simulink library "xrbsDSP_r3"  (Simulink 5.0)
undefined symbols (not defined in the file or in its folder): FIR1, Ft, mem
libraries: xbsIndex_r3 x329
(part 3 of 4)

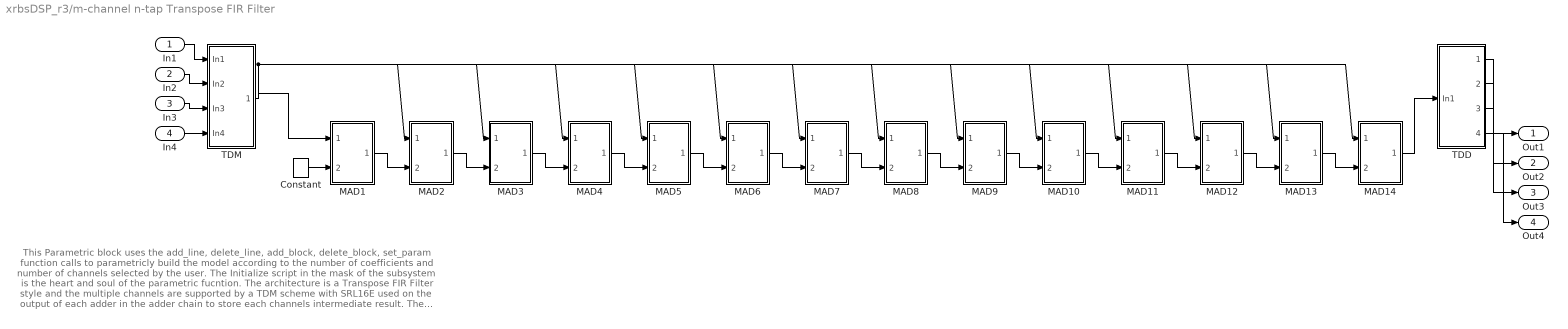
== system xrbsDSP_r3/m-channel n-tap Transpose FIR Filter ==
  note: This Parametric block uses the add_line, delete_line, add_block, delete_block, set_param function calls to parametricly
      | build the model according to the number of coefficients and number of channels selected by the user. The Initialize script in
      | the mask of the subsystem is the heart and soul of the parametric fucntion.
      |
      | The architecture is a Transpose FIR Filter style and the multiple channels are supported by a TDM scheme with SRL16E used
      | on the output of each adder in the adder chain to store each channels intermediate result. The clock will always be N channels
      | times faster that the input sample rate.
  In1 : Inport
  In2 : Inport  Port=2
  In3 : Inport  Port=3
  In4 : Inport  Port=4
  Constant : xbsIndex_r3/Constant  const=0  arith_type=Unsigned  n_bits=1  bin_pt=0  explicit_period=off  period=1  dbl_ovrd=off
  MAD1 : Subsystem  mask(MAD Block){coef=coef_array(1), coef_bitwidth=coef_bitwidth, coef_binpt=coef_binpt, channels=channels}
      mask prompts: coef "Coefficient Value"; coef_bitwidth "Coefficient Bit Width"; coef_binpt "Coefficient Binary Point"; channels "Number of Channels"
  MAD10 : Subsystem  mask(MAD Block){coef=coef_array(10), coef_bitwidth=coef_bitwidth, coef_binpt=coef_binpt, channels=channels}
      mask prompts: coef "Coefficient Value"; coef_bitwidth "Coefficient Bit Width"; coef_binpt "Coefficient Binary Point"; channels "Number of Channels"
  MAD11 : Subsystem  mask(MAD Block){coef=coef_array(11), coef_bitwidth=coef_bitwidth, coef_binpt=coef_binpt, channels=channels}
      mask prompts: coef "Coefficient Value"; coef_bitwidth "Coefficient Bit Width"; coef_binpt "Coefficient Binary Point"; channels "Number of Channels"
  MAD12 : Subsystem  mask(MAD Block){coef=coef_array(12), coef_bitwidth=coef_bitwidth, coef_binpt=coef_binpt, channels=channels}
      mask prompts: coef "Coefficient Value"; coef_bitwidth "Coefficient Bit Width"; coef_binpt "Coefficient Binary Point"; channels "Number of Channels"
  MAD13 : Subsystem  mask(MAD Block){coef=coef_array(13), coef_bitwidth=coef_bitwidth, coef_binpt=coef_binpt, channels=channels}
      mask prompts: coef "Coefficient Value"; coef_bitwidth "Coefficient Bit Width"; coef_binpt "Coefficient Binary Point"; channels "Number of Channels"
  MAD14 : Subsystem  mask(MAD Block){coef=coef_array(14), coef_bitwidth=coef_bitwidth, coef_binpt=coef_binpt, channels=channels}
      mask prompts: coef "Coefficient Value"; coef_bitwidth "Coefficient Bit Width"; coef_binpt "Coefficient Binary Point"; channels "Number of Channels"
  MAD2 : Subsystem  mask(MAD Block){coef=coef_array(2), coef_bitwidth=coef_bitwidth, coef_binpt=coef_binpt, channels=channels}
      mask prompts: coef "Coefficient Value"; coef_bitwidth "Coefficient Bit Width"; coef_binpt "Coefficient Binary Point"; channels "Number of Channels"
  MAD3 : Subsystem  mask(MAD Block){coef=coef_array(3), coef_bitwidth=coef_bitwidth, coef_binpt=coef_binpt, channels=channels}
      mask prompts: coef "Coefficient Value"; coef_bitwidth "Coefficient Bit Width"; coef_binpt "Coefficient Binary Point"; channels "Number of Channels"
  MAD4 : Subsystem  mask(MAD Block){coef=coef_array(4), coef_bitwidth=coef_bitwidth, coef_binpt=coef_binpt, channels=channels}
      mask prompts: coef "Coefficient Value"; coef_bitwidth "Coefficient Bit Width"; coef_binpt "Coefficient Binary Point"; channels "Number of Channels"
  MAD5 : Subsystem  mask(MAD Block){coef=coef_array(5), coef_bitwidth=coef_bitwidth, coef_binpt=coef_binpt, channels=channels}
      mask prompts: coef "Coefficient Value"; coef_bitwidth "Coefficient Bit Width"; coef_binpt "Coefficient Binary Point"; channels "Number of Channels"
  MAD6 : Subsystem  mask(MAD Block){coef=coef_array(6), coef_bitwidth=coef_bitwidth, coef_binpt=coef_binpt, channels=channels}
      mask prompts: coef "Coefficient Value"; coef_bitwidth "Coefficient Bit Width"; coef_binpt "Coefficient Binary Point"; channels "Number of Channels"
  MAD7 : Subsystem  mask(MAD Block){coef=coef_array(7), coef_bitwidth=coef_bitwidth, coef_binpt=coef_binpt, channels=channels}
      mask prompts: coef "Coefficient Value"; coef_bitwidth "Coefficient Bit Width"; coef_binpt "Coefficient Binary Point"; channels "Number of Channels"
  MAD8 : Subsystem  mask(MAD Block){coef=coef_array(8), coef_bitwidth=coef_bitwidth, coef_binpt=coef_binpt, channels=channels}
      mask prompts: coef "Coefficient Value"; coef_bitwidth "Coefficient Bit Width"; coef_binpt "Coefficient Binary Point"; channels "Number of Channels"
  MAD9 : Subsystem  mask(MAD Block){coef=coef_array(9), coef_bitwidth=coef_bitwidth, coef_binpt=coef_binpt, channels=channels}
      mask prompts: coef "Coefficient Value"; coef_bitwidth "Coefficient Bit Width"; coef_binpt "Coefficient Binary Point"; channels "Number of Channels"
  TDD : Subsystem
      mask Type: TDD
      mask Description: Multi-Channel Time Division DeMultiplexer
  TDM : Subsystem
  Out1 : Outport
  Out2 : Outport  Port=2
  Out3 : Outport  Port=3
  Out4 : Outport  Port=4
  wires:
  Constant/1 -> MAD1/2(In2)
  TDM/1(Out1) -> MAD1/1(In1), MAD2/1(In1), MAD3/1(In1), MAD4/1(In1), MAD5/1(In1), MAD6/1(In1), MAD7/1(In1), MAD8/1(In1), MAD9/1(In1), MAD10/1(In1), MAD11/1(In1), MAD12/1(In1), MAD13/1(In1), MAD14/1(In1)
  In1/1 -> TDM/1(In1)
  MAD1/1(Out1) -> MAD2/2(In2)
  MAD2/1(Out1) -> MAD3/2(In2)
  MAD3/1(Out1) -> MAD4/2(In2)
  MAD4/1(Out1) -> MAD5/2(In2)
  MAD5/1(Out1) -> MAD6/2(In2)
  MAD6/1(Out1) -> MAD7/2(In2)
  MAD7/1(Out1) -> MAD8/2(In2)
  MAD8/1(Out1) -> MAD9/2(In2)
  MAD9/1(Out1) -> MAD10/2(In2)
  MAD10/1(Out1) -> MAD11/2(In2)
  MAD11/1(Out1) -> MAD12/2(In2)
  MAD12/1(Out1) -> MAD13/2(In2)
  MAD13/1(Out1) -> MAD14/2(In2)
  MAD14/1(Out1) -> TDD/1(In1)
  TDD/1(Out1) -> Out1/1
  TDD/2(Out2) -> Out2/1
  TDD/3(Out3) -> Out3/1
  TDD/4(Out4) -> Out4/1
  In2/1 -> TDM/2(In2)
  In3/1 -> TDM/3(In3)
  In4/1 -> TDM/4(In4)

== system xrbsDSP_r3/n-tap Dual Port Memory MAC FIR Filter ==
  note: The 'Address Control' subsystem
      | provides the necessary address
      | logic for the Dual Port RAM.
      | The control logic creates a cyclic
      | RAM buffer for port A (data buffer)
      | to create the required shifting
      | effect.
  note: A Dual Port Block RAM implements the input data buffer.
      | The address port runs n times faster than the data port,
      | where n is the number of filter taps.
      |
      | The filter coefficients are also stored in the same Dual Port
      | Block RAM and are output from port B.
  note: A down sampler reduces the capture register
      | sample period to the output sample period.
      | The block is configured with latency to obtain  the
      | most efficient hardware implementation.  The down
      | sampling rate is equal to the coefficient array length.
  note: A capture register is required for streaming
      | operation, since the MAC engine reloads its
      | accumulator with an incoming sample after
      | computing the last partial product for an output
      | sample.
  note: As configured, the filter occupies 84 slices, 1 dedicated multiplier,
      | and 1 block memory.  The maximum clock frequency is approximately
      | 180 MHz in a Xilinx xc2vp2-7 part (advanced speeds files 1.69, ISE
      | 5.1.03i software).
  din : Inport
  Accumulator : xbsIndex_r3/Accumulator  n_bits=accum_bit_width  overflow=Wrap  operation=Add  scale=1  explicit_period=off  period=1  rst=on  hasbypass=on  en=off  dbl_ovrd=off  show_param=off  gen_core=on  use_rpm=off
      settings: xl_area=[0, 0, 0, 0, 0, 0, 0]
  Address Control : Subsystem
  Capture Register : xbsIndex_r3/Register  init=0  reg_only_valid=on  explicit_period=off  period=1  rst=off  en=on  out_en=off  dbl_ovrd=off  show_param=off
      settings: xl_area=[0, 0, 0, 0, 0, 0, 0]
  Delay : xbsIndex_r3/Delay  latency=3  reg_retiming=off  explicit_period=off  period=1  en=off  accept_only_valid=off  init_zero=on  dbl_ovrd=off  show_param=off
      settings: xl_area=[0, 0, 0, 0, 0, 0, 0]
  Down Sample : xbsIndex_r3/Down Sample  sample_ratio=length(coef)  sample_phase="Last Value of Frame  (most efficient)"  latency=1  en=off  dbl_ovrd=off  show_param=off
      settings: xl_area=[0, 0, 0, 0, 0, 0, 0]
  Dual Port RAM : Subsystem
  Mult : xbsIndex_r3/Mult  precision=Full  arith_type="Signed  (2's comp)"  n_bits=8  bin_pt=2  quantization=Truncate  overflow=Wrap  latency=2  explicit_period=off  period=1/(22050*length(coef))  en=off  dbl_ovrd=off  show_param=off  mult_type=Parallel  oversample=2  use_embedded=on  pipeline=on  use_rpm=off  placement_style=Rectangular Shape  gen_core=on
      settings: xl_area=[0, 0, 0, 0, 0, 0, 0]
  dout : Outport
  wires:
  Delay/1 -> Accumulator/2, Capture Register/2
  Address Control/4(rst) -> Delay/1
  Dual Port RAM/2(dout_b) -> Mult/2
  Dual Port RAM/1(dout_a) -> Mult/1
  din/1 -> Dual Port RAM/1(din)
  Address Control/3(coef_addr) -> Dual Port RAM/4(coef_addr)
  Address Control/2(we) -> Dual Port RAM/3(we)
  Address Control/1(data_addr) -> Dual Port RAM/2(data_addr)
  Capture Register/1 -> Down Sample/1
  Accumulator/1 -> Capture Register/1
  Down Sample/1 -> dout/1
  Mult/1 -> Accumulator/1

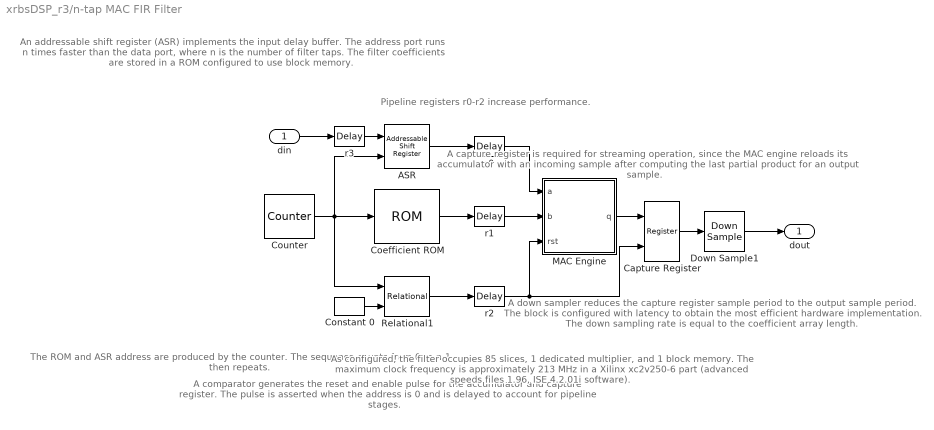
== system xrbsDSP_r3/n-tap MAC FIR Filter ==
  note: A capture register is required for streaming
      | operation, since the MAC engine reloads its
      | accumulator with an incoming sample after
      | computing the last partial product for an output
      | sample.
  note: Pipeline registers r0-r2
      | increase performance.
  note: An addressable shift register (ASR)
      | implements the input delay buffer.
      | The address port runs n times faster
      | than the data port, where n is the number
      | of filter taps.
      |
      | The filter coefficients are stored in a ROM
      | configured to use block memory.
  note: The ROM and ASR
      | address are produced
      | by the counter.  The
      | sequence counts from
      | 0 to n-1, then repeats.
  note: A comparator generates
      | the reset and enable
      | pulse for the accumulator
      | and capture register.  The
      | pulse is asserted when
      | the address is 0 and is
      | delayed to account for
      | pipeline stages.
  note: As configured, the  filter occupies 85 slices, 1 dedicated multiplier, and
      | 1 block memory.  The maximum clock frequency is approximately
      | 213 MHz in a Xilinx xc2v250-6 part (advanced speeds files 1.96, ISE
      | 4.2.01i software).
  note: A down sampler reduces the capture register
      | sample period to the output sample period.
      | The block is configured with latency to obtain  the
      | most efficient hardware implementation.  The down
      | sampling rate is equal to the coefficient array length.
  din : Inport
  ASR : xbsIndex_r3/Addressable Shift Register  infer_latency=on  depth=2  initVector=0  explicit_period=off  period=1  accept_only_valid=off  en=off  dbl_ovrd=off  show_param=off  use_rpm=off  gen_core=off
      settings: xl_area=[0, 0, 0, 0, 0, 0, 0]
  Capture Register : xbsIndex_r3/Register  init=0  reg_only_valid=on  explicit_period=off  period=1  rst=off  en=on  out_en=off  dbl_ovrd=off  show_param=off
      settings: xl_area=[0, 0, 0, 0, 0, 0, 0]
  Coefficient ROM : xbsIndex_r3/ROM  depth=length(coef)  initVector=coef  arith_type="Signed  (2's comp)"  n_bits=coef_n_bits  bin_pt=coef_bin_pt  latency=1  init_zero=on  explicit_period=off  period=1  rst=off  init_reg=0  en=off  dbl_ovrd=off  show_param=off  distributed_mem=off  use_rpm=off  gen_core=on
      settings: xl_area=[0, 0, 0, 0, 0, 0, 0]
  Constant 0 : xbsIndex_r3/Constant  const=0  arith_type=Unsigned  n_bits=1  bin_pt=0  explicit_period=off  period=1  dbl_ovrd=off
  Counter : xbsIndex_r3/Counter  cnt_type=Count Limited  n_bits=ceil(log2(length(coef)))  bin_pt=0  arith_type=Unsigned  start_count=0  cnt_to=length(coef)-1  cnt_by_val=1  operation=Up  explicit_period=on  period=smpl_period/length(coef)  load_pin=off  rst=off  en=off  dbl_ovrd=off  show_param=off  use_rpm=on  gen_core=on
      settings: xl_area=[0, 0, 0, 0, 0, 0, 0]
  Down Sample1 : xbsIndex_r3/Down Sample  sample_ratio=length(coef)  sample_phase="Last Value of Frame  (most efficient)"  latency=1  en=off  dbl_ovrd=off  show_param=off
      settings: xl_area=[0, 0, 0, 0, 0, 0, 0]
  MAC Engine : Subsystem
  Relational1 : xbsIndex_r3/Relational  mode=a=b  latency=3  explicit_period=off  period=1  en=off  dbl_ovrd=off  show_param=off
      settings: xl_area=[0, 0, 0, 0, 0, 0, 0]
  r0 : xbsIndex_r3/Delay  latency=2  reg_retiming=off  explicit_period=off  period=1  en=off  accept_only_valid=off  init_zero=on  dbl_ovrd=off  show_param=off
      settings: xl_area=[0, 0, 0, 0, 0, 0, 0]
  r1 : xbsIndex_r3/Delay  latency=1  reg_retiming=off  explicit_period=off  period=1  en=off  accept_only_valid=off  init_zero=on  dbl_ovrd=off  show_param=off
      settings: xl_area=[0, 0, 0, 0, 0, 0, 0]
  r2 : xbsIndex_r3/Delay  latency=1  reg_retiming=off  explicit_period=off  period=1  en=off  accept_only_valid=off  init_zero=on  dbl_ovrd=off  show_param=off
      settings: xl_area=[0, 0, 0, 0, 0, 0, 0]
  r3 : xbsIndex_r3/Delay  latency=1  reg_retiming=off  explicit_period=off  period=1  en=off  accept_only_valid=off  init_zero=on  dbl_ovrd=off  show_param=off
      settings: xl_area=[0, 0, 0, 0, 0, 0, 0]
  dout : Outport
  wires:
  din/1 -> r3/1
  r1/1 -> MAC Engine/2(b)
  r0/1 -> MAC Engine/1(a)
  ASR/1 -> r0/1
  Counter/1 -> Coefficient ROM/1, ASR/2, Relational1/1
  r3/1 -> ASR/1
  Constant 0/1 -> Relational1/2
  Coefficient ROM/1 -> r1/1
  MAC Engine/1(q) -> Capture Register/1
  Down Sample1/1 -> dout/1
  Capture Register/1 -> Down Sample1/1
  Relational1/1 -> r2/1
  r2/1 -> Capture Register/2, MAC Engine/3(rst)

== system xrbsDSP_r3/2 Channel  Decimate by 2  MAC FIR Filter/2 Channel Accum ==
  d : Inport
  rst : Inport  Port=2
  AddSub : xbsIndex_r3/AddSub  mode=Addition  precision=User Defined  arith_type="Signed  (2's comp)"  n_bits=ceil(log2(coef_sum*(2^(bit_width-1))))+1  bin_pt=coef_bin_pt+bin_pt  quantization=Truncate  overflow=Wrap  latency=0  explicit_period=on  period=-1  use_carryin=off  use_carryout=off  en=off  dbl_ovrd=off  show_param=off  use_core=on  pipeline=off  use_rpm=off  gen_core=on
      settings: xl_area=[18 0 0 36 0 0 0]
  Delay : xbsIndex_r3/Delay  Orientation=left  latency=1  reg_retiming=off  explicit_period=off  period=1  en=off  accept_only_valid=off  init_zero=on  dbl_ovrd=off  show_param=off
      settings: xl_area=[18 36 0 0 0 0 0]
  Mux : xbsIndex_r3/Mux  inputs=2  precision=Full  arith_type="Signed  (2's comp)"  n_bits=8  bin_pt=2  quantization=Truncate  overflow=Wrap  latency=0  explicit_period=off  period=1  en=off  dbl_ovrd=off  show_param=off  mux_type=off  use_rpm=off  gen_core=on
      settings: xl_area=[36 0 0 36 0 0 0]
  Register : xbsIndex_r3/Register  init=0  reg_only_valid=off  explicit_period=off  period=1  rst=off  en=off  out_en=off  dbl_ovrd=off  show_param=off
      settings: xl_area=[18 36 0 0 0 0 0]
  q : Outport
  wires:
  Delay/1 -> AddSub/2
  Register/1 -> q/1, Delay/1
  Mux/1 -> Register/1
  AddSub/1 -> Mux/3
  rst/1 -> Mux/1
  d/1 -> Mux/2, AddSub/1

== system xrbsDSP_r3/2 Channel  Decimate by 2  MAC FIR Filter/2:1 Mux ==
  din1 : Inport
  din2 : Inport  Port=2
  Counter : xbsIndex_r3/Counter  cnt_type=Free Running  n_bits=1  bin_pt=0  arith_type=Unsigned  start_count=0  cnt_to=Inf  cnt_by_val=1  operation=Up  explicit_period=off  period=Ts/2  load_pin=off  rst=off  en=off  dbl_ovrd=off  use_rpm=off  gen_core=on
      settings: xl_area=[2 1 0 1 0 0 0]
  Delay2 : xbsIndex_r3/Delay  latency=1  reg_retiming=off  explicit_period=off  period=1  en=off  accept_only_valid=off  init_zero=on  dbl_ovrd=off
      settings: xl_area=[0, 0, 0, 0, 0, 0, 0]
  Mux : xbsIndex_r3/Mux  inputs=2  precision=Full  arith_type="Signed  (2's comp)"  n_bits=8  bin_pt=2  quantization=Truncate  overflow=Wrap  latency=0  mux_type=off  explicit_period=off  period=1  en=off  dbl_ovrd=off  use_rpm=off  gen_core=on
      settings: xl_area=[0, 0, 0, 0, 0, 0, 0]
  Up Sample : xbsIndex_r3/Up Sample  sample_ratio=2  copy_samples=on  dbl_ovrd=off
      settings: xl_area=[0, 0, 0, 0, 0, 0, 0]
  Up Sample1 : xbsIndex_r3/Up Sample  sample_ratio=2  copy_samples=on  dbl_ovrd=off
      settings: xl_area=[0, 0, 0, 0, 0, 0, 0]
  Up Sample2 : xbsIndex_r3/Up Sample  sample_ratio=length(coef)/4  copy_samples=on  dbl_ovrd=off
      settings: xl_area=[0, 0, 0, 0, 0, 0, 0]
  dout : Outport
  wires:
  Up Sample2/1 -> dout/1
  din2/1 -> Up Sample1/1
  din1/1 -> Up Sample/1
  Delay2/1 -> Up Sample2/1
  Mux/1 -> Delay2/1
  Counter/1 -> Mux/1
  Up Sample1/1 -> Mux/3
  Up Sample/1 -> Mux/2

== system xrbsDSP_r3/2 Channel  Decimate by 2  MAC FIR Filter/Accum Control ==
  Constant1 : xbsIndex_r3/Constant  const=2  arith_type=Unsigned  n_bits=2  bin_pt=0  explicit_period=off  period=1  dbl_ovrd=off
  Constant4 : xbsIndex_r3/Constant  const=0  arith_type=Unsigned  n_bits=2  bin_pt=0  explicit_period=off  period=1  dbl_ovrd=off
  Constant5 : xbsIndex_r3/Constant  const=1  arith_type=Unsigned  n_bits=2  bin_pt=0  explicit_period=off  period=1  dbl_ovrd=off
  Counter : xbsIndex_r3/Counter  cnt_type=Free Running  n_bits=2  bin_pt=0  arith_type=Unsigned  start_count=0  cnt_to=Inf  cnt_by_val=1  operation=Up  explicit_period=off  period=Ts/2  load_pin=off  rst=off  en=off  dbl_ovrd=off  use_rpm=off  gen_core=on
      settings: xl_area=[1 2 0 2 0 0 0]
  Logical : xbsIndex_r3/Logical  logical_function=OR  inputs=2  precision=Full  arith_type=Unsigned  n_bits=8  bin_pt=2  align_bp=on  latency=0  explicit_period=off  period=1  en=off  dbl_ovrd=off
      settings: xl_area=[1 0 0 1 0 0 0]
  Relational1 : xbsIndex_r3/Relational  mode=a=b  latency=0  explicit_period=off  period=1  en=off  dbl_ovrd=off
      settings: xl_area=[2 0 0 1 0 0 0]
  Relational4 : xbsIndex_r3/Relational  mode=a=b  latency=0  explicit_period=off  period=1  en=off  dbl_ovrd=off
      settings: xl_area=[2 0 0 1 0 0 0]
  Relational5 : xbsIndex_r3/Relational  mode=a=b  latency=0  explicit_period=off  period=1  en=off  dbl_ovrd=off
      settings: xl_area=[2 0 0 1 0 0 0]
  rst : Outport
  en_a : Outport  Port=2
  en_b : Outport  Port=3
  wires:
  Relational1/1 -> en_b/1
  Constant1/1 -> Relational1/2
  Logical/1 -> rst/1
  Relational5/1 -> en_a/1, Logical/2
  Relational4/1 -> Logical/1
  Constant5/1 -> Relational5/2
  Constant4/1 -> Relational4/2
  Counter/1 -> Relational4/1, Relational1/1, Relational5/1

== system xrbsDSP_r3/2 Channel  Decimate by 2  MAC FIR Filter/Data Buffer ==
  din : Inport
  data_addr : Inport  Port=2
  en : Inport  Port=3
  coef_addr : Inport  Port=4
  ASR : xbsIndex_r3/Addressable Shift Register  infer_latency=on  depth=2  initVector=[0]  explicit_period=off  period=1  accept_only_valid=off  en=on  dbl_ovrd=off  use_rpm=off  gen_core=<empty>
      settings: xl_area=[0, 0, 0, 0, 0, 0, 0]
  Delay1 : xbsIndex_r3/Delay  latency=1  reg_retiming=off  explicit_period=off  period=1  en=off  accept_only_valid=off  init_zero=on  dbl_ovrd=off
      settings: xl_area=[0, 0, 0, 0, 0, 0, 0]
  ROM : xbsIndex_r3/ROM  depth=length(coef)  initVector=coef  arith_type="Signed  (2's comp)"  n_bits=coef_bit_width  bin_pt=coef_bin_pt  latency=1  distributed_mem=off  init_zero=on  explicit_period=off  period=1  rst=off  init_reg=0  en=off  dbl_ovrd=off  use_rpm=off  gen_core=on
      settings: xl_area=[0, 0, 0, 0, 0, 0, 0]
  dout : Outport
  coef_out : Outport  Port=2
  wires:
  Delay1/1 -> dout/1
  ROM/1 -> coef_out/1
  coef_addr/1 -> ROM/1
  ASR/1 -> Delay1/1
  data_addr/1 -> ASR/2
  din/1 -> ASR/1
  en/1 -> ASR/3

== system xrbsDSP_r3/2 Channel  Decimate by 2  MAC FIR Filter/Memory Control ==
  Addr Counter : xbsIndex_r3/Counter  cnt_type=Count Limited  n_bits=ceil(log2(length(coef)-1))  bin_pt=0  arith_type=Unsigned  start_count=0  cnt_to=length(coef)-4  cnt_by_val=4  operation=Up  explicit_period=off  period=Ts/(length(coef)/2)  load_pin=off  rst=off  en=off  dbl_ovrd=off  use_rpm=off  gen_core=on
      settings: xl_area=[0, 0, 0, 0, 0, 0, 0]
  Coef Counter : xbsIndex_r3/Counter  cnt_type=Count Limited  n_bits=ceil(log2(length(coef)-1))  bin_pt=0  arith_type=Unsigned  start_count=0  cnt_to=length(coef)-1  cnt_by_val=1  operation=Up  explicit_period=off  period=Ts/(length(coef)/2)  load_pin=off  rst=off  en=off  dbl_ovrd=off  use_rpm=off  gen_core=on
      settings: xl_area=[0, 0, 0, 0, 0, 0, 0]
  Constant : xbsIndex_r3/Constant  const=length(coef)-4  arith_type=Unsigned  n_bits=ceil(log2(length(coef)-4))  bin_pt=0  explicit_period=off  period=1  dbl_ovrd=off
  Relational : xbsIndex_r3/Relational  mode=a=b  latency=0  explicit_period=off  period=1  en=off  dbl_ovrd=off
      settings: xl_area=[0, 0, 0, 0, 0, 0, 0]
  data_addr : Outport
  we : Outport  Port=2
  coef_addr : Outport  Port=3
  wires:
  Coef Counter/1 -> coef_addr/1
  Relational/1 -> we/1
  Constant/1 -> Relational/2
  Addr Counter/1 -> data_addr/1, Relational/1

== system xrbsDSP_r3/2n+1-tap Linear Phase  MAC FIR Filter/MAC Engine ==
  note: This subsystem implements a multiply-accumulate engine.
  a : Inport
  b : Inport  Port=2
  rst : Inport  Port=3
  Accumulator : xbsIndex_r3/Accumulator  n_bits=ceil(log2(max(1,sum(abs(coef*2^coef_bin_pt)))))+smpl_n_bits + 1  overflow=Wrap  operation=Add  scale=1  explicit_period=off  period=1  rst=on  hasbypass=on  en=off  dbl_ovrd=off  show_param=off  gen_core=on  use_rpm=off
      settings: xl_area=[0, 0, 0, 0, 0, 0, 0]
  Mult : xbsIndex_r3/Mult  precision=User Defined  arith_type="Signed  (2's comp)"  n_bits=max(ceil(log2(max(1,max(abs(coef*2^coef_bin_pt)))))+smpl_n_bits + 1,smpl_bin_pt+coef_bin_pt)  bin_pt=smpl_bin_pt+coef_bin_pt  quantization=Truncate  overflow=Wrap  latency=2  explicit_period=off  period=1  en=off  dbl_ovrd=off  show_param=off  mult_type=Parallel  oversample=2  use_embedded=on  pipeline=on  use_rpm=on  placement_style=Rectangular Shape  gen_core=on
      settings: xl_area=[0, 0, 0, 0, 0, 0, 0]
  q : Outport
  wires:
  rst/1 -> Accumulator/2
  b/1 -> Mult/2
  Accumulator/1 -> q/1
  a/1 -> Mult/1
  Mult/1 -> Accumulator/1

== system xrbsDSP_r3/2n-tap Linear Phase  MAC FIR Filter/MAC Engine ==
  note: This subsystem implements a multiply-accumulate engine.
  a : Inport
  b : Inport  Port=2
  rst : Inport  Port=3
  Accumulator : xbsIndex_r3/Accumulator  n_bits=ceil(log2(max(1,sum(abs(coef*2^coef_bin_pt)))))+smpl_n_bits + 1  overflow=Wrap  operation=Add  scale=1  explicit_period=off  period=1  rst=on  hasbypass=on  en=off  dbl_ovrd=off  show_param=off  gen_core=on  use_rpm=off
      settings: xl_area=[0, 0, 0, 0, 0, 0, 0]
  Mult : xbsIndex_r3/Mult  precision=User Defined  arith_type="Signed  (2's comp)"  n_bits=max(ceil(log2(max(1,max(abs(coef*2^coef_bin_pt)))))+smpl_n_bits + 1,smpl_bin_pt+coef_bin_pt)  bin_pt=smpl_bin_pt+coef_bin_pt  quantization=Truncate  overflow=Wrap  latency=2  explicit_period=off  period=1  en=off  dbl_ovrd=off  show_param=off  mult_type=Parallel  oversample=2  use_embedded=on  pipeline=on  use_rpm=on  placement_style=Rectangular Shape  gen_core=on
      settings: xl_area=[0, 0, 0, 0, 0, 0, 0]
  q : Outport
  wires:
  Mult/1 -> Accumulator/1
  a/1 -> Mult/1
  Accumulator/1 -> q/1
  b/1 -> Mult/2
  rst/1 -> Accumulator/2

== system xrbsDSP_r3/4n-tap  MAC FIR Filter/4-Input  Adder Tree ==
  a1 : Inport
  b1 : Inport  Port=2
  a2 : Inport  Port=3
  b2 : Inport  Port=4
  AddSub1 : xbsIndex_r3/AddSub  mode=Addition  precision=Full  arith_type=Unsigned  n_bits=8  bin_pt=2  quantization=Truncate  overflow=Wrap  latency=1  explicit_period=off  period=1  en=off  dbl_ovrd=off  use_core=on  gen_core=on  pipeline=off  use_rpm=off
      settings: xl_area=[0, 0, 0, 0, 0, 0, 0]
  AddSub2 : xbsIndex_r3/AddSub  mode=Addition  precision=Full  arith_type=Unsigned  n_bits=8  bin_pt=2  quantization=Truncate  overflow=Wrap  latency=1  explicit_period=off  period=1  en=off  dbl_ovrd=off  use_core=on  gen_core=on  pipeline=off  use_rpm=off
      settings: xl_area=[0, 0, 0, 0, 0, 0, 0]
  AddSub3 : xbsIndex_r3/AddSub  mode=Addition  precision=Full  arith_type=Unsigned  n_bits=8  bin_pt=2  quantization=Truncate  overflow=Wrap  latency=1  explicit_period=off  period=1  en=off  dbl_ovrd=off  use_core=on  gen_core=on  pipeline=off  use_rpm=off
      settings: xl_area=[0, 0, 0, 0, 0, 0, 0]
  dout : Outport
  wires:
  AddSub1/1 -> AddSub3/1
  AddSub2/1 -> AddSub3/2
  a1/1 -> AddSub1/1
  b1/1 -> AddSub1/2
  AddSub3/1 -> dout/1
  a2/1 -> AddSub2/1
  b2/1 -> AddSub2/2

== system xrbsDSP_r3/CIC Filter/Differentiator1 ==
  In1 : Inport
  AddSub : xbsIndex_r3/AddSub  mode=Subtraction  precision=User Defined  arith_type="Signed  (2's comp)"  n_bits=output_bitwidth  bin_pt=output_binpt  quantization=Truncate  overflow=Wrap  latency=1  explicit_period=off  period=1  use_carryin=off  use_carryout=off  en=off  dbl_ovrd=off  show_param=off  use_core=on  pipeline=off  use_rpm=on  gen_core=on
      settings: xl_area=[53 106 0 106 0 0 0]
  Delay : xbsIndex_r3/Delay  latency=m  reg_retiming=off  explicit_period=off  period=1  en=off  accept_only_valid=off  init_zero=on  dbl_ovrd=off  show_param=off
      settings: xl_area=[53 106 0 0 0 0 0]
  Out1 : Outport
  wires:
  In1/1 -> Delay/1, AddSub/1
  AddSub/1 -> Out1/1
  Delay/1 -> AddSub/2

== system xrbsDSP_r3/CIC Filter/Differentiator2 ==
  In1 : Inport
  AddSub : xbsIndex_r3/AddSub  mode=Subtraction  precision=User Defined  arith_type="Signed  (2's comp)"  n_bits=output_bitwidth  bin_pt=output_binpt  quantization=Truncate  overflow=Wrap  latency=1  explicit_period=off  period=1  use_carryin=off  use_carryout=off  en=off  dbl_ovrd=off  show_param=off  use_core=on  pipeline=off  use_rpm=on  gen_core=on
      settings: xl_area=[53 106 0 106 0 0 0]
  Delay : xbsIndex_r3/Delay  latency=m  reg_retiming=off  explicit_period=off  period=1  en=off  accept_only_valid=off  init_zero=on  dbl_ovrd=off  show_param=off
      settings: xl_area=[53 106 0 0 0 0 0]
  Out1 : Outport
  wires:
  Delay/1 -> AddSub/2
  AddSub/1 -> Out1/1
  In1/1 -> AddSub/1, Delay/1

== system xrbsDSP_r3/CIC Filter/Differentiator3 ==
  In1 : Inport
  AddSub : xbsIndex_r3/AddSub  mode=Subtraction  precision=User Defined  arith_type="Signed  (2's comp)"  n_bits=output_bitwidth  bin_pt=output_binpt  quantization=Truncate  overflow=Wrap  latency=1  explicit_period=off  period=1  use_carryin=off  use_carryout=off  en=off  dbl_ovrd=off  show_param=off  use_core=on  pipeline=off  use_rpm=on  gen_core=on
      settings: xl_area=[53 106 0 106 0 0 0]
  Delay : xbsIndex_r3/Delay  latency=m  reg_retiming=off  explicit_period=off  period=1  en=off  accept_only_valid=off  init_zero=on  dbl_ovrd=off  show_param=off
      settings: xl_area=[53 106 0 0 0 0 0]
  Out1 : Outport
  wires:
  Delay/1 -> AddSub/2
  AddSub/1 -> Out1/1
  In1/1 -> AddSub/1, Delay/1

== system xrbsDSP_r3/CIC Filter/Integrator1 ==
  In1 : Inport
  Accumulator : xbsIndex_r3/Accumulator  n_bits=output_bitwidth  overflow=Wrap  operation=Add  scale=1  explicit_period=off  period=1  rst=off  hasbypass=off  en=off  dbl_ovrd=off  show_param=off  gen_core=on  use_rpm=on
      settings: xl_area=[53 106 0 106 0 0 0]
  Out1 : Outport
  wires:
  In1/1 -> Accumulator/1
  Accumulator/1 -> Out1/1

== system xrbsDSP_r3/CIC Filter/Integrator2 ==
  In1 : Inport
  Accumulator : xbsIndex_r3/Accumulator  n_bits=output_bitwidth  overflow=Wrap  operation=Add  scale=1  explicit_period=off  period=1  rst=off  hasbypass=off  en=off  dbl_ovrd=off  show_param=off  gen_core=on  use_rpm=on
      settings: xl_area=[53 106 0 106 0 0 0]
  Out1 : Outport
  wires:
  Accumulator/1 -> Out1/1
  In1/1 -> Accumulator/1

== system xrbsDSP_r3/CIC Filter/Integrator3 ==
  In1 : Inport
  Accumulator : xbsIndex_r3/Accumulator  n_bits=output_bitwidth  overflow=Wrap  operation=Add  scale=1  explicit_period=off  period=1  rst=off  hasbypass=off  en=off  dbl_ovrd=off  show_param=off  gen_core=on  use_rpm=on
      settings: xl_area=[53 106 0 106 0 0 0]
  Out1 : Outport
  wires:
  Accumulator/1 -> Out1/1
  In1/1 -> Accumulator/1

== system xrbsDSP_r3/Dual Port Memory Interpolation MAC FIR Filter/Address Control ==
  note: The lowest counter, 'Data_Counter2,' is used to create a
      | reset/capture signal for the accumulator. This signal goes
      | high N times (interpolation rate) for every new sample that
      | is loaded in the filter.
  note: The coefficent counter controls the enable
      | on the data counter. This ensures the cyclic
      | RAM Buffer effect in the data section of the
      |  memory.
  Coef_Counter : xbsIndex_r3/Counter  Priority=5  cnt_type=Count Limited  n_bits=ceil(log2((length(coef)-1)+length(coef)/ir))  bin_pt=0  arith_type=Unsigned  start_count=length(coef)/ir  cnt_to=(length(coef)-1)+length(coef)/ir  cnt_by_val=1  operation=Up  explicit_period=off  period=Ts/length(coef)  load_pin=off  rst=off  en=off  dbl_ovrd=off  use_rpm=on  gen_core=on
      settings: xl_area=[5 7 0 9 0 0 0]
  Constant1 : xbsIndex_r3/Constant  const=(length(coef)-1)+length(coef)/ir  arith_type=Unsigned  n_bits=ceil(log2((length(coef)-1)+length(coef)/ir))  bin_pt=0  explicit_period=off  period=1  dbl_ovrd=off
  Constant2 : xbsIndex_r3/Constant  const=length(coef)/ir-1  arith_type=Unsigned  n_bits=ceil(log2((length(coef)-1)+length(coef)/ir))  bin_pt=0  explicit_period=off  period=1  dbl_ovrd=off
  Data_Counter1 : xbsIndex_r3/Counter  Priority=5  cnt_type=Count Limited  n_bits=ceil(log2((length(coef)-1)+length(coef)/ir))  bin_pt=0  arith_type=Unsigned  start_count=0  cnt_to=length(coef)/ir-1  cnt_by_val=1  operation=Up  explicit_period=off  period=Ft/length(coef)  load_pin=off  rst=off  en=on  dbl_ovrd=off  use_rpm=on  gen_core=on
      settings: xl_area=[5 7 0 9 0 0 0]
  Data_Counter2 : xbsIndex_r3/Counter  Priority=5  cnt_type=Count Limited  n_bits=ceil(log2((length(coef)-1)+length(coef)/ir))  bin_pt=0  arith_type=Unsigned  start_count=0  cnt_to=length(coef)/ir-1  cnt_by_val=1  operation=Up  explicit_period=off  period=Ts/length(coef)  load_pin=off  rst=off  en=off  dbl_ovrd=off  use_rpm=on  gen_core=on
      settings: xl_area=[5 7 0 9 0 0 0]
  Delay : xbsIndex_r3/Delay  latency=1  reg_retiming=off  explicit_period=off  period=1  en=off  accept_only_valid=off  init_zero=on  dbl_ovrd=off
      settings: xl_area=[1 1 0 0 0 0 0]
  Inverter : xbsIndex_r3/Inverter  Orientation=left  latency=0  explicit_period=off  period=1  en=off  dbl_ovrd=off
      settings: xl_area=[1 0 0 1 0 0 0]
  Relational1 : xbsIndex_r3/Relational  mode=a=b  latency=0  explicit_period=off  period=1  en=off  dbl_ovrd=off
      settings: xl_area=[2 0 0 4 0 0 0]
  Relational2 : xbsIndex_r3/Relational  mode=a=b  latency=0  explicit_period=off  period=1  en=off  dbl_ovrd=off
      settings: xl_area=[2 0 0 4 0 0 0]
  data_addr : Outport
  we : Outport  Port=2
  coef_addr : Outport  Port=3
  reset : Outport  Port=4
  wires:
  Relational2/1 -> reset/1
  Constant2/1 -> Relational2/2
  Data_Counter2/1 -> Relational2/1
  Relational1/1 -> Delay/1, Inverter/1
  Constant1/1 -> Relational1/2
  Inverter/1 -> Data_Counter1/1
  Delay/1 -> we/1
  Data_Counter1/1 -> data_addr/1
  Coef_Counter/1 -> coef_addr/1, Relational1/1

== system xrbsDSP_r3/Dual Port Memory Interpolation MAC FIR Filter/Dual Port RAM ==
  data_A : Inport
  addr_A : Inport  Port=2
  we_A : Inport  Port=3
  addr_B : Inport  Port=4
  Convert : xbsIndex_r3/Convert  arith_type="Signed  (2's comp)"  n_bits=coef_bit_width  bin_pt=coef_bin_pt  quantization=Truncate  overflow=Wrap  latency=0  explicit_period=off  period=1  dbl_ovrd=off  inserted_by_tool=off
      settings: xl_area=[0 0 0 0 0 0 0]
  Dual Port RAM : xbsIndex_r3/Dual Port RAM  depth=length([zeros(1, length(coef)/ir) coef(:)'])  initVector=[zeros(1, length(coef)/ir) coef(:)']  write_mode_A=Read After Write  write_mode_B=Read After Write  latency=1  distributed_mem=off  mem_collision=off  init_zero=on  explicit_period=off  period=1  dbl_ovrd=off  rst_a=off  init_a=0  rst_b=off  init_b=0  use_rpm=off  gen_core=on
      settings: xl_area=[0 0 1 0 0 0 0]
  Up Sample : xbsIndex_r3/Up Sample  sample_ratio=no_taps  copy_samples=on  dbl_ovrd=off
      settings: xl_area=[0 0 0 0 0 0 0]
  Zero : xbsIndex_r3/Constant  Priority=5  const=0  arith_type="Signed  (2's comp)"  n_bits=coef_bit_width + coef_pad_bits  bin_pt=coef_bin_pt  explicit_period=off  period=Ft/length(coef)  dbl_ovrd=off
  Zero1 : xbsIndex_r3/Constant  Priority=5  const=0  arith_type=Boolean  n_bits=1  bin_pt=0  explicit_period=off  period=Ft/length(coef)  dbl_ovrd=off
  pad : Subsystem
  unpad : Subsystem
  dout_A : Outport
  dout_B : Outport  Port=2
  wires:
  Convert/1 -> dout_B/1
  Up Sample/1 -> pad/1(din)
  pad/1(dout) -> Dual Port RAM/2
  addr_B/1 -> Dual Port RAM/4
  we_A/1 -> Dual Port RAM/3
  unpad/1(dout) -> dout_A/1
  addr_A/1 -> Dual Port RAM/1
  data_A/1 -> Up Sample/1
  Dual Port RAM/1 -> unpad/1(din)
  Zero1/1 -> Dual Port RAM/6
  Zero/1 -> Dual Port RAM/5
  Dual Port RAM/2 -> Convert/1

== system xrbsDSP_r3/Interpolation Filter/Adder Tree ==
  din1 : Inport
  din2 : Inport  Port=2
  din3 : Inport  Port=3
  din4 : Inport  Port=4
  AddSub : xbsIndex_r3/AddSub  mode=Addition  precision=Full  arith_type=Unsigned  n_bits=8  bin_pt=2  quantization=Truncate  overflow=Wrap  latency=1  explicit_period=off  period=1  en=off  dbl_ovrd=off  use_core=off  pipeline=off  use_rpm=off  gen_core=off
      settings: xl_area=[0, 0, 0, 0, 0, 0, 0]
  AddSub1 : xbsIndex_r3/AddSub  mode=Addition  precision=Full  arith_type=Unsigned  n_bits=8  bin_pt=2  quantization=Truncate  overflow=Wrap  latency=1  explicit_period=off  period=1  en=off  dbl_ovrd=off  use_core=off  pipeline=off  use_rpm=off  gen_core=off
      settings: xl_area=[0, 0, 0, 0, 0, 0, 0]
  AddSub2 : xbsIndex_r3/AddSub  mode=Addition  precision=Full  arith_type=Unsigned  n_bits=8  bin_pt=2  quantization=Truncate  overflow=Wrap  latency=1  explicit_period=off  period=1  en=off  dbl_ovrd=off  use_core=off  pipeline=off  use_rpm=off  gen_core=off
      settings: xl_area=[0, 0, 0, 0, 0, 0, 0]
  sum : Outport
  wires:
  din4/1 -> AddSub1/2
  din3/1 -> AddSub1/1
  AddSub2/1 -> sum/1
  din2/1 -> AddSub/2
  din1/1 -> AddSub/1
  AddSub1/1 -> AddSub2/2
  AddSub/1 -> AddSub2/1

== system xrbsDSP_r3/Interpolation Filter/Coef Buffer ==
  addr : Inport
  ROM : xbsIndex_r3/ROM  depth=length(mem(1,:))  initVector=mem(1,:)  arith_type="Signed  (2's comp)"  n_bits=coef_bit_width  bin_pt=coef_bin_pt  latency=1  distributed_mem=off  init_zero=on  explicit_period=off  period=1  rst=off  init_reg=0  en=off  dbl_ovrd=off  use_rpm=off  gen_core=on
      settings: xl_area=[0, 0, 0, 0, 0, 0, 0]
  ROM1 : xbsIndex_r3/ROM  depth=length(mem(2,:))  initVector=mem(2,:)  arith_type="Signed  (2's comp)"  n_bits=coef_bit_width  bin_pt=coef_bin_pt  latency=1  distributed_mem=off  init_zero=on  explicit_period=off  period=1  rst=off  init_reg=0  en=off  dbl_ovrd=off  use_rpm=off  gen_core=on
      settings: xl_area=[0, 0, 0, 0, 0, 0, 0]
  ROM2 : xbsIndex_r3/ROM  depth=length(mem(3,:))  initVector=mem(3,:)  arith_type="Signed  (2's comp)"  n_bits=coef_bit_width  bin_pt=coef_bin_pt  latency=1  distributed_mem=off  init_zero=on  explicit_period=off  period=1  rst=off  init_reg=0  en=off  dbl_ovrd=off  use_rpm=off  gen_core=on
      settings: xl_area=[0, 0, 0, 0, 0, 0, 0]
  ROM3 : xbsIndex_r3/ROM  depth=length(mem(4,:))  initVector=mem(4,:)  arith_type="Signed  (2's comp)"  n_bits=coef_bit_width  bin_pt=coef_bin_pt  latency=1  distributed_mem=off  init_zero=on  explicit_period=off  period=1  rst=off  init_reg=0  en=off  dbl_ovrd=off  use_rpm=off  gen_core=on
      settings: xl_area=[0, 0, 0, 0, 0, 0, 0]
  coef0 : Outport
  coef1 : Outport  Port=2
  coef2 : Outport  Port=3
  coef3 : Outport  Port=4
  wires:
  addr/1 -> ROM3/1, ROM2/1, ROM1/1, ROM/1
  ROM3/1 -> coef3/1
  ROM2/1 -> coef2/1
  ROM1/1 -> coef1/1
  ROM/1 -> coef0/1

== system xrbsDSP_r3/Interpolation Filter/Control ==
  0:x_SRL_depth-1 : xbsIndex_r3/Counter  cnt_type=Count Limited  n_bits=ceil(log2(x_SRL_depth))  bin_pt=0  arith_type=Unsigned  start_count=0  cnt_to=x_SRL_depth-1  cnt_by_val=1  operation=Up  explicit_period=off  period=T_clock  load_pin=off  rst=off  en=off  dbl_ovrd=off  use_rpm=off  gen_core=on
      settings: xl_area=[0, 0, 0, 0, 0, 0, 0]
  Concat : xbsIndex_r3/Concat  num_inputs=2  explicit_period=off  period=1  dbl_ovrd=off
  Constant : xbsIndex_r3/Constant  const=x_SRL_depth-1  arith_type=Unsigned  n_bits=ceil(log2(x_SRL_depth))  bin_pt=0  explicit_period=off  period=1  dbl_ovrd=off
  Constant1 : xbsIndex_r3/Constant  const=interp_ratio-1  arith_type=Unsigned  n_bits=ceil(log2(interp_ratio))  bin_pt=0  explicit_period=off  period=1  dbl_ovrd=off
  Counter : xbsIndex_r3/Counter  cnt_type=Free Running  n_bits=ceil(log2(interp_ratio))  bin_pt=0  arith_type=Unsigned  start_count=interp_ratio-1  cnt_to=Inf  cnt_by_val=1  operation=Up  explicit_period=off  period=1  load_pin=off  rst=off  en=on  dbl_ovrd=off  use_rpm=off  gen_core=on
      settings: xl_area=[0, 0, 0, 0, 0, 0, 0]
  Logical : xbsIndex_r3/Logical  logical_function=AND  inputs=2  precision=Full  arith_type=Unsigned  n_bits=8  bin_pt=2  align_bp=off  latency=0  explicit_period=off  period=1  en=off  dbl_ovrd=off
      settings: xl_area=[0, 0, 0, 0, 0, 0, 0]
  Relational : xbsIndex_r3/Relational  mode=a=b  latency=0  explicit_period=off  period=1  en=off  dbl_ovrd=off
      settings: xl_area=[0, 0, 0, 0, 0, 0, 0]
  Relational1 : xbsIndex_r3/Relational  mode=a=b  latency=0  explicit_period=off  period=1  en=off  dbl_ovrd=off
      settings: xl_area=[0, 0, 0, 0, 0, 0, 0]
  data_addr : Outport
  result : Outport  Port=2
  coef_addr : Outport  Port=3
  srl16_we : Outport  Port=4
  wires:
  Constant1/1 -> Relational1/2
  Relational1/1 -> Logical/2
  Logical/1 -> result/1
  Concat/1 -> coef_addr/1
  Counter/1 -> Concat/1, Relational1/1
  Constant/1 -> Relational/2
  0:x_SRL_depth-1/1 -> data_addr/1, Concat/2, Relational/1
  Relational/1 -> Counter/1, srl16_we/1, Logical/1

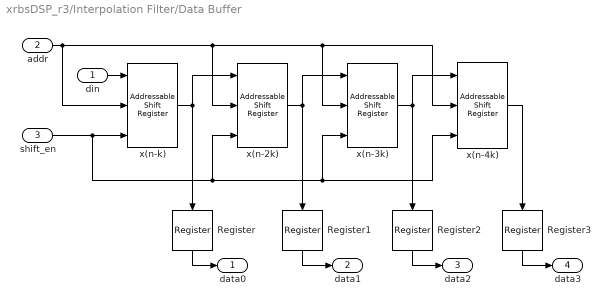
== system xrbsDSP_r3/Interpolation Filter/Data Buffer ==
  din : Inport
  addr : Inport  Port=2
  shift_en : Inport  Port=3
  Register{,1..3} (4 alike) : xbsIndex_r3/Register  Orientation=down  init=0  reg_only_valid=off  explicit_period=off  period=1  rst=off  en=off  out_en=off  dbl_ovrd=off
      settings: xl_area=[0, 0, 0, 0, 0, 0, 0]
  x(n-2k) : xbsIndex_r3/Addressable Shift Register  infer_latency=off  depth=x_SRL_depth  initVector=[0]  explicit_period=off  period=1  accept_only_valid=off  en=on  dbl_ovrd=off  use_rpm=off  gen_core=<empty>
      settings: xl_area=[0, 0, 0, 0, 0, 0, 0]
  x(n-3k) : xbsIndex_r3/Addressable Shift Register  infer_latency=off  depth=x_SRL_depth  initVector=[0]  explicit_period=off  period=1  accept_only_valid=off  en=on  dbl_ovrd=off  use_rpm=off  gen_core=<empty>
      settings: xl_area=[0, 0, 0, 0, 0, 0, 0]
  x(n-4k) : xbsIndex_r3/Addressable Shift Register  infer_latency=off  depth=x_SRL_depth  initVector=[0]  explicit_period=off  period=1  accept_only_valid=off  en=on  dbl_ovrd=off  use_rpm=off  gen_core=<empty>
      settings: xl_area=[0, 0, 0, 0, 0, 0, 0]
  x(n-k) : xbsIndex_r3/Addressable Shift Register  infer_latency=off  depth=x_SRL_depth  initVector=[0]  explicit_period=off  period=1  accept_only_valid=off  en=on  dbl_ovrd=off  use_rpm=off  gen_core=<empty>
      settings: xl_area=[0, 0, 0, 0, 0, 0, 0]
  data0 : Outport
  data1 : Outport  Port=2
  data2 : Outport  Port=3
  data3 : Outport  Port=4
  wires:
  Register3/1 -> data3/1
  Register2/1 -> data2/1
  Register1/1 -> data1/1
  Register/1 -> data0/1
  x(n-4k)/1 -> Register3/1
  x(n-3k)/1 -> Register2/1, x(n-4k)/1
  x(n-2k)/1 -> x(n-3k)/1, Register1/1
  x(n-k)/1 -> Register/1, x(n-2k)/1
  shift_en/1 -> x(n-4k)/3, x(n-3k)/3, x(n-2k)/3, x(n-k)/3
  addr/1 -> x(n-4k)/2, x(n-3k)/2, x(n-2k)/2, x(n-k)/2
  din/1 -> x(n-k)/1

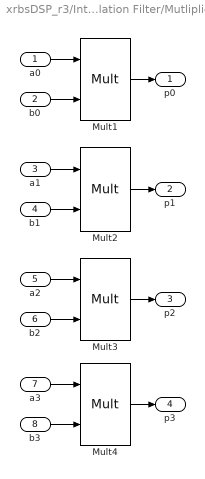
== system xrbsDSP_r3/Interpolation Filter/Mutlipliers ==
  a0 : Inport
  b0 : Inport  Port=2
  a1 : Inport  Port=3
  b1 : Inport  Port=4
  a2 : Inport  Port=5
  b2 : Inport  Port=6
  a3 : Inport  Port=7
  b3 : Inport  Port=8
  Mult{1..4} (4 alike) : xbsIndex_r3/Mult  precision=Full  arith_type="Signed  (2's comp)"  n_bits=8  bin_pt=2  quantization=Truncate  overflow=Wrap  latency=1  explicit_period=off  period=1  en=off  dbl_ovrd=off  show_param=off  mult_type=Parallel  oversample=2  use_embedded=on  pipeline=on  use_rpm=off  placement_style=Rectangular Shape  gen_core=on
      settings: xl_area=[0, 0, 0, 0, 0, 0, 0]
  p0 : Outport
  p1 : Outport  Port=2
  p2 : Outport  Port=3
  p3 : Outport  Port=4
  wires:
  Mult4/1 -> p3/1
  Mult3/1 -> p2/1
  Mult2/1 -> p1/1
  Mult1/1 -> p0/1
  b3/1 -> Mult4/2
  a3/1 -> Mult4/1
  b2/1 -> Mult3/2
  a2/1 -> Mult3/1
  b1/1 -> Mult2/2
  a1/1 -> Mult2/1
  b0/1 -> Mult1/2
  a0/1 -> Mult1/1

== system xrbsDSP_r3/m-channel n-tap Transpose FIR Filter/MAD1 ==
  In1 : Inport
  In2 : Inport  Port=2
  AddSub : xbsIndex_r3/AddSub  mode=Addition  precision=User Defined  arith_type="Signed  (2's comp)"  n_bits=output_bitwidth  bin_pt=output_binpt  quantization=Truncate  overflow=Wrap  latency=channels  explicit_period=off  period=1  use_carryin=off  use_carryout=off  en=off  dbl_ovrd=off  show_param=off  use_core=on  pipeline=off  use_rpm=off  gen_core=on
      settings: xl_area=[32 64 0 49 0 0 0]
  Constant : xbsIndex_r3/Constant  const=coef  arith_type="Signed  (2's comp)"  n_bits=coef_bitwidth  bin_pt=coef_binpt  explicit_period=off  period=1  dbl_ovrd=off
  Mult : xbsIndex_r3/Mult  precision=Full  arith_type="Signed  (2's comp)"  n_bits=8  bin_pt=2  quantization=Truncate  overflow=Wrap  latency=2  explicit_period=off  period=1  en=off  dbl_ovrd=off  show_param=off  mult_type=Parallel  oversample=2  use_embedded=on  pipeline=on  use_rpm=off  placement_style=Rectangular Shape  gen_core=on
      settings: xl_area=[17 34 0 0 0 1 0]
  Out1 : Outport
  wires:
  Mult/1 -> AddSub/1
  Constant/1 -> Mult/2
  In1/1 -> Mult/1
  AddSub/1 -> Out1/1
  In2/1 -> AddSub/2

== system xrbsDSP_r3/m-channel n-tap Transpose FIR Filter/MAD10 ==
  In1 : Inport
  In2 : Inport  Port=2
  AddSub : xbsIndex_r3/AddSub  mode=Addition  precision=User Defined  arith_type="Signed  (2's comp)"  n_bits=output_bitwidth  bin_pt=output_binpt  quantization=Truncate  overflow=Wrap  latency=channels  explicit_period=off  period=1  use_carryin=off  use_carryout=off  en=off  dbl_ovrd=off  show_param=off  use_core=on  pipeline=off  use_rpm=off  gen_core=on
      settings: xl_area=[32 64 0 64 0 0 0]
  Constant : xbsIndex_r3/Constant  const=coef  arith_type="Signed  (2's comp)"  n_bits=coef_bitwidth  bin_pt=coef_binpt  explicit_period=off  period=1  dbl_ovrd=off
  Mult : xbsIndex_r3/Mult  precision=Full  arith_type="Signed  (2's comp)"  n_bits=8  bin_pt=2  quantization=Truncate  overflow=Wrap  latency=2  explicit_period=off  period=1  en=off  dbl_ovrd=off  show_param=off  mult_type=Parallel  oversample=2  use_embedded=on  pipeline=on  use_rpm=off  placement_style=Rectangular Shape  gen_core=on
      settings: xl_area=[17 34 0 0 0 1 0]
  Out1 : Outport
  wires:
  In2/1 -> AddSub/2
  AddSub/1 -> Out1/1
  In1/1 -> Mult/1
  Constant/1 -> Mult/2
  Mult/1 -> AddSub/1

== system xrbsDSP_r3/m-channel n-tap Transpose FIR Filter/MAD11 ==
  In1 : Inport
  In2 : Inport  Port=2
  AddSub : xbsIndex_r3/AddSub  mode=Addition  precision=User Defined  arith_type="Signed  (2's comp)"  n_bits=output_bitwidth  bin_pt=output_binpt  quantization=Truncate  overflow=Wrap  latency=channels  explicit_period=off  period=1  use_carryin=off  use_carryout=off  en=off  dbl_ovrd=off  show_param=off  use_core=on  pipeline=off  use_rpm=off  gen_core=on
      settings: xl_area=[32 64 0 64 0 0 0]
  Constant : xbsIndex_r3/Constant  const=coef  arith_type="Signed  (2's comp)"  n_bits=coef_bitwidth  bin_pt=coef_binpt  explicit_period=off  period=1  dbl_ovrd=off
  Mult : xbsIndex_r3/Mult  precision=Full  arith_type="Signed  (2's comp)"  n_bits=8  bin_pt=2  quantization=Truncate  overflow=Wrap  latency=2  explicit_period=off  period=1  en=off  dbl_ovrd=off  show_param=off  mult_type=Parallel  oversample=2  use_embedded=on  pipeline=on  use_rpm=off  placement_style=Rectangular Shape  gen_core=on
      settings: xl_area=[17 34 0 0 0 1 0]
  Out1 : Outport
  wires:
  In2/1 -> AddSub/2
  AddSub/1 -> Out1/1
  In1/1 -> Mult/1
  Constant/1 -> Mult/2
  Mult/1 -> AddSub/1

== system xrbsDSP_r3/m-channel n-tap Transpose FIR Filter/MAD12 ==
  In1 : Inport
  In2 : Inport  Port=2
  AddSub : xbsIndex_r3/AddSub  mode=Addition  precision=User Defined  arith_type="Signed  (2's comp)"  n_bits=output_bitwidth  bin_pt=output_binpt  quantization=Truncate  overflow=Wrap  latency=channels  explicit_period=off  period=1  use_carryin=off  use_carryout=off  en=off  dbl_ovrd=off  show_param=off  use_core=on  pipeline=off  use_rpm=off  gen_core=on
      settings: xl_area=[32 64 0 64 0 0 0]
  Constant : xbsIndex_r3/Constant  const=coef  arith_type="Signed  (2's comp)"  n_bits=coef_bitwidth  bin_pt=coef_binpt  explicit_period=off  period=1  dbl_ovrd=off
  Mult : xbsIndex_r3/Mult  precision=Full  arith_type="Signed  (2's comp)"  n_bits=8  bin_pt=2  quantization=Truncate  overflow=Wrap  latency=2  explicit_period=off  period=1  en=off  dbl_ovrd=off  show_param=off  mult_type=Parallel  oversample=2  use_embedded=on  pipeline=on  use_rpm=off  placement_style=Rectangular Shape  gen_core=on
      settings: xl_area=[17 34 0 0 0 1 0]
  Out1 : Outport
  wires:
  In2/1 -> AddSub/2
  AddSub/1 -> Out1/1
  In1/1 -> Mult/1
  Constant/1 -> Mult/2
  Mult/1 -> AddSub/1

== system xrbsDSP_r3/m-channel n-tap Transpose FIR Filter/MAD13 ==
  In1 : Inport
  In2 : Inport  Port=2
  AddSub : xbsIndex_r3/AddSub  mode=Addition  precision=User Defined  arith_type="Signed  (2's comp)"  n_bits=output_bitwidth  bin_pt=output_binpt  quantization=Truncate  overflow=Wrap  latency=channels  explicit_period=off  period=1  use_carryin=off  use_carryout=off  en=off  dbl_ovrd=off  show_param=off  use_core=on  pipeline=off  use_rpm=off  gen_core=on
      settings: xl_area=[32 64 0 64 0 0 0]
  Constant : xbsIndex_r3/Constant  const=coef  arith_type="Signed  (2's comp)"  n_bits=coef_bitwidth  bin_pt=coef_binpt  explicit_period=off  period=1  dbl_ovrd=off
  Mult : xbsIndex_r3/Mult  precision=Full  arith_type="Signed  (2's comp)"  n_bits=8  bin_pt=2  quantization=Truncate  overflow=Wrap  latency=2  explicit_period=off  period=1  en=off  dbl_ovrd=off  show_param=off  mult_type=Parallel  oversample=2  use_embedded=on  pipeline=on  use_rpm=off  placement_style=Rectangular Shape  gen_core=on
      settings: xl_area=[17 34 0 0 0 1 0]
  Out1 : Outport
  wires:
  In2/1 -> AddSub/2
  AddSub/1 -> Out1/1
  In1/1 -> Mult/1
  Constant/1 -> Mult/2
  Mult/1 -> AddSub/1

== system xrbsDSP_r3/m-channel n-tap Transpose FIR Filter/MAD14 ==
  In1 : Inport
  In2 : Inport  Port=2
  AddSub : xbsIndex_r3/AddSub  mode=Addition  precision=User Defined  arith_type="Signed  (2's comp)"  n_bits=output_bitwidth  bin_pt=output_binpt  quantization=Truncate  overflow=Wrap  latency=channels  explicit_period=off  period=1  use_carryin=off  use_carryout=off  en=off  dbl_ovrd=off  show_param=off  use_core=on  pipeline=off  use_rpm=off  gen_core=on
      settings: xl_area=[32 64 0 64 0 0 0]
  Constant : xbsIndex_r3/Constant  const=coef  arith_type="Signed  (2's comp)"  n_bits=coef_bitwidth  bin_pt=coef_binpt  explicit_period=off  period=1  dbl_ovrd=off
  Mult : xbsIndex_r3/Mult  precision=Full  arith_type="Signed  (2's comp)"  n_bits=8  bin_pt=2  quantization=Truncate  overflow=Wrap  latency=2  explicit_period=off  period=1  en=off  dbl_ovrd=off  show_param=off  mult_type=Parallel  oversample=2  use_embedded=on  pipeline=on  use_rpm=off  placement_style=Rectangular Shape  gen_core=on
      settings: xl_area=[17 34 0 0 0 1 0]
  Out1 : Outport
  wires:
  In2/1 -> AddSub/2
  AddSub/1 -> Out1/1
  In1/1 -> Mult/1
  Constant/1 -> Mult/2
  Mult/1 -> AddSub/1

== system xrbsDSP_r3/m-channel n-tap Transpose FIR Filter/MAD2 ==
  In1 : Inport
  In2 : Inport  Port=2
  AddSub : xbsIndex_r3/AddSub  mode=Addition  precision=User Defined  arith_type="Signed  (2's comp)"  n_bits=output_bitwidth  bin_pt=output_binpt  quantization=Truncate  overflow=Wrap  latency=channels  explicit_period=off  period=1  use_carryin=off  use_carryout=off  en=off  dbl_ovrd=off  show_param=off  use_core=on  pipeline=off  use_rpm=off  gen_core=on
      settings: xl_area=[32 64 0 64 0 0 0]
  Constant : xbsIndex_r3/Constant  const=coef  arith_type="Signed  (2's comp)"  n_bits=coef_bitwidth  bin_pt=coef_binpt  explicit_period=off  period=1  dbl_ovrd=off
  Mult : xbsIndex_r3/Mult  precision=Full  arith_type="Signed  (2's comp)"  n_bits=8  bin_pt=2  quantization=Truncate  overflow=Wrap  latency=2  explicit_period=off  period=1  en=off  dbl_ovrd=off  show_param=off  mult_type=Parallel  oversample=2  use_embedded=on  pipeline=on  use_rpm=off  placement_style=Rectangular Shape  gen_core=on
      settings: xl_area=[17 34 0 0 0 1 0]
  Out1 : Outport
  wires:
  In2/1 -> AddSub/2
  AddSub/1 -> Out1/1
  In1/1 -> Mult/1
  Constant/1 -> Mult/2
  Mult/1 -> AddSub/1

== system xrbsDSP_r3/m-channel n-tap Transpose FIR Filter/MAD3 ==
  In1 : Inport
  In2 : Inport  Port=2
  AddSub : xbsIndex_r3/AddSub  mode=Addition  precision=User Defined  arith_type="Signed  (2's comp)"  n_bits=output_bitwidth  bin_pt=output_binpt  quantization=Truncate  overflow=Wrap  latency=channels  explicit_period=off  period=1  use_carryin=off  use_carryout=off  en=off  dbl_ovrd=off  show_param=off  use_core=on  pipeline=off  use_rpm=off  gen_core=on
      settings: xl_area=[32 64 0 64 0 0 0]
  Constant : xbsIndex_r3/Constant  const=coef  arith_type="Signed  (2's comp)"  n_bits=coef_bitwidth  bin_pt=coef_binpt  explicit_period=off  period=1  dbl_ovrd=off
  Mult : xbsIndex_r3/Mult  precision=Full  arith_type="Signed  (2's comp)"  n_bits=8  bin_pt=2  quantization=Truncate  overflow=Wrap  latency=2  explicit_period=off  period=1  en=off  dbl_ovrd=off  show_param=off  mult_type=Parallel  oversample=2  use_embedded=on  pipeline=on  use_rpm=off  placement_style=Rectangular Shape  gen_core=on
      settings: xl_area=[17 34 0 0 0 1 0]
  Out1 : Outport
  wires:
  In2/1 -> AddSub/2
  AddSub/1 -> Out1/1
  In1/1 -> Mult/1
  Constant/1 -> Mult/2
  Mult/1 -> AddSub/1
